simulink model "SEDC_DC_Motor_APP"  (R2022b)
settings: Solver=VariableStepAuto  StartTime=0.0  StopTime=10.0  MaxStep=1e-3  RelTol=1e-3
values from neighbouring files (symbols this model uses):
  Kphi = 1.6    [DC_motor_SEDC.m]
  TL = 20    [DC_motor_SEDC.m]
  Va = 160    [DC_motor_SEDC.m]
settings Model: Creator=Abanob_Sameh  LastModifiedBy=Abanob_Sameh

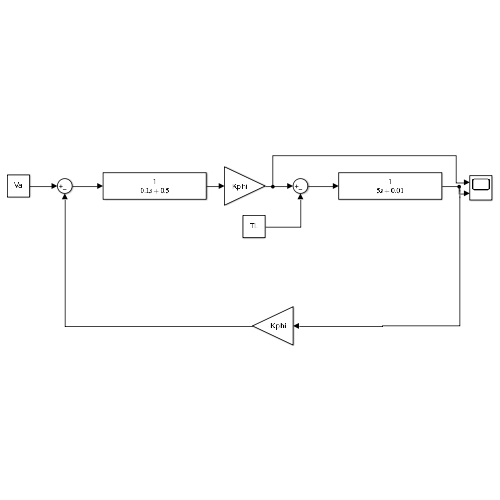
[thumbnail: Simulink's stored preview of the top-level diagram]
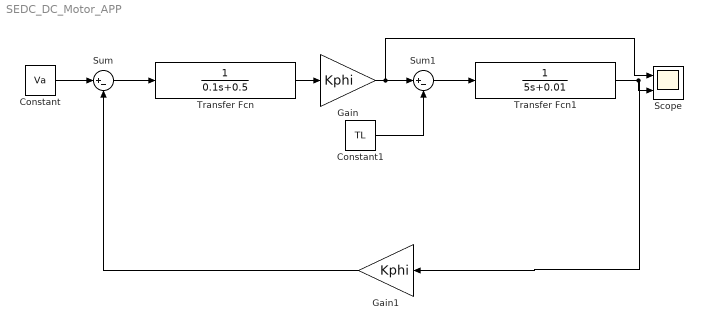
== system SEDC_DC_Motor_APP ==
  Constant : Constant  Value=Va
  Constant1 : Constant  Value=TL
  Gain : Gain  Gain=Kphi
  Gain1 : Gain  Gain=Kphi
  Scope : Scope  NumInputPorts=2
  Sum : Sum  Inputs=|+-
  Sum1 : Sum  Inputs=|+-
  Transfer Fcn : TransferFcn  Denominator=[0.1 0.5]
  Transfer Fcn1 : TransferFcn  Denominator=[5 0.01]
  wires:
  Constant/1 -> Sum/1
  Transfer Fcn/1 -> Gain/1
  Sum/1 -> Transfer Fcn/1
  Gain/1 -> Scope/1, Sum1/1
  Sum1/1 -> Transfer Fcn1/1
  Constant1/1 -> Sum1/2
  Transfer Fcn1/1 -> Gain1/1, Scope/2
  Gain1/1 -> Sum/2
